simulink model "Model"  (R2020a)
settings: Solver=VariableStepAuto  StartTime=0.0  StopTime=3  RelTol=1e-3
values from neighbouring files (symbols this model uses):
  A = [0 1 0 0 ... (first row only)    [Inverted_Pendulum_and_Cart.m]
  B = [0; -m*l/z; 0; (J+m*l^2)/z]    [Inverted_Pendulum_and_Cart.m]
  K = place(A,B,pol_Des)    [Inverted_Pendulum_and_Cart.m]
settings Model: EnablePacing=on  Creator=sabir  LastModifiedBy=sabir

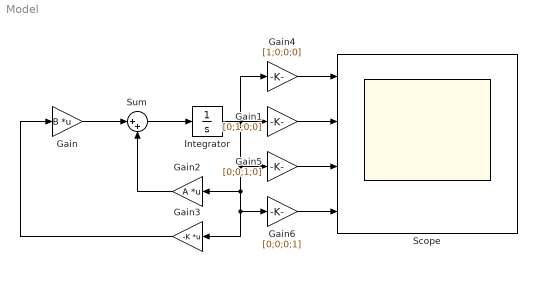
== system Model ==
  Gain : Gain  Gain=B  Multiplication=Matrix(K*u)
  Gain1 : Gain  Gain=[0;1;0;0]
  Gain2 : Gain  Gain=A  Multiplication=Matrix(K*u)
  Gain3 : Gain  Gain=-K  Multiplication=Matrix(K*u)
  Gain4 : Gain  Gain=[1;0;0;0]
  Gain5 : Gain  Gain=[0;0;1;0]
  Gain6 : Gain  Gain=[0;0;0;1]
  Integrator : Integrator  InitialCondition=[0.05;0;0;0]
  Scope : Scope  NumInputPorts=4
  Sum : Sum  Inputs=|++
  wires:
  Gain2/1 -> Sum/2
  Gain/1 -> Sum/1
  Gain3/1 -> Gain/1
  Sum/1 -> Integrator/1
  Integrator/1 -> Gain4/1, Gain5/1, Gain2/1, Gain6/1, Gain3/1, Gain1/1
  Gain4/1 -> Scope/1
  Gain1/1 -> Scope/2
  Gain5/1 -> Scope/3
  Gain6/1 -> Scope/4
